simulink library "tenneco_lib"  (R2016b)
settings: Solver=ode45  StartTime=0.0  StopTime=10.0  RelTol=1e-3
undefined symbols (not defined in the file): Com_cntAMBInitTO_c, Com_cntAMBStopTO_c, Com_cntEC1InitTO_c, Com_cntEC1StopTO_c, Com_swAMBRx_c, Com_swEC1Rx_c, Com_swUseSPN108_c, Com_swUseSPN543_c, const, Env_pAmbPDflt_c, Env_pAmbPKOff_c, Env_pAmbPOvrd_c, Env_swAmbPOvrd_c, MSG_INIT_TIMEOUT, MSG_NOT_RECEIVED, MSG_RECEIVED_NOW, MSG_STOP_TIMEOUT
libraries: simulink x19, tenneco_lib x2
(part 5 of 5)

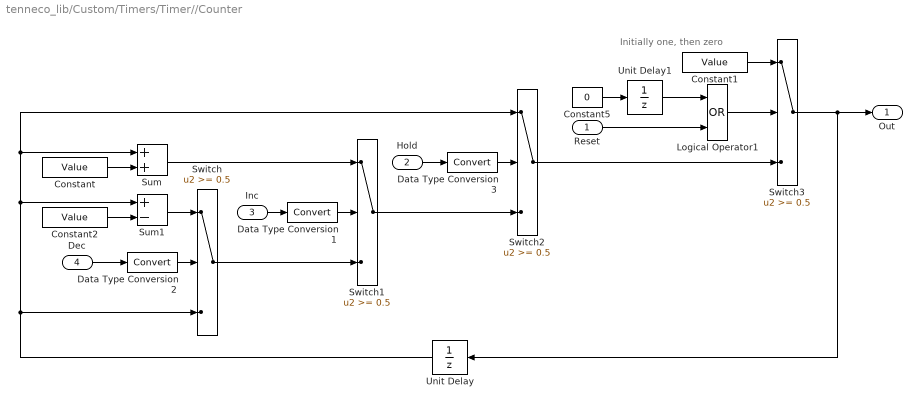
== system tenneco_lib/Custom/Timers/Timer//Counter ==
  note: Initially one,
      | then zero
  Reset : Inport  mask(Standard Inport){Port=1}
      mask prompts: Port "Simulink:blkprm_prompts:InOutportPortNum"
      mask help: Provide an input port for subsystems.
      mask TypeOptions Port: Port
  Hold : Inport  Port=2  mask(Standard Inport){Port=2}
      mask prompts: Port "Simulink:blkprm_prompts:InOutportPortNum"
      mask help: Provide an input port for subsystems.
      mask TypeOptions Port: Port
  Inc : Inport  Port=3  mask(Standard Inport){Port=3}
      mask prompts: Port "Simulink:blkprm_prompts:InOutportPortNum"
      mask help: Provide an input port for subsystems.
      mask TypeOptions Port: Port
  Dec : Inport  Port=4  mask(Standard Inport){Port=4}
      mask prompts: Port "Simulink:blkprm_prompts:InOutportPortNum"
      mask help: Provide an input port for subsystems.
      mask TypeOptions Port: Port
  Constant : Constant  Value=Value  mask(Constant){Value=INC_STEP}
      mask prompts: Value "Simulink:blkprm_prompts:ConstConstValue"
      mask help: Output the constant specified by the 'Constant value' parameter. If 'Constant value' is a vector, treat the constant value as a 1-D array.
      mask init: same as tenneco_lib/Custom/Logical/Latch/Constant
      mask TypeOptions Value: Value
      mask Display: disp(str)
  Constant1 : Constant  Value=Value  mask(Constant){Value=INIT}
      mask prompts: Value "Simulink:blkprm_prompts:ConstConstValue"
      mask help: Output the constant specified by the 'Constant value' parameter. If 'Constant value' is a vector, treat the constant value as a 1-D array.
      mask init: same as tenneco_lib/Custom/Logical/Latch/Constant
      mask TypeOptions Value: Value
      mask Display: disp(str)
  Constant2 : Constant  Value=Value  mask(Constant){Value=DEC_STEP}
      mask prompts: Value "Simulink:blkprm_prompts:ConstConstValue"
      mask help: Output the constant specified by the 'Constant value' parameter. If 'Constant value' is a vector, treat the constant value as a 1-D array.
      mask init: same as tenneco_lib/Custom/Logical/Latch/Constant
      mask TypeOptions Value: Value
      mask Display: disp(str)
  Constant5 : Constant  Value=0  OutDataTypeStr=Inherit: Inherit via back propagation
  Data Type Conversion1 : DataTypeConversion  mask(Data Type Conversion){OutDataTypeStr=Inherit: Inherit via back propagation}
      mask prompts: OutDataTypeStr "Simulink:blkprm_prompts:OUTPUT_UNIFIEDDATATYPE"
      mask help: Convert the input to the data type and scaling of the output.
      mask TypeOptions OutDataTypeStr: OutDataTypeStr
  Data Type Conversion2 : DataTypeConversion  mask(Data Type Conversion){OutDataTypeStr=Inherit: Inherit via back propagation}
      mask prompts: OutDataTypeStr "Simulink:blkprm_prompts:OUTPUT_UNIFIEDDATATYPE"
      mask help: Convert the input to the data type and scaling of the output.
      mask TypeOptions OutDataTypeStr: OutDataTypeStr
  Data Type Conversion3 : DataTypeConversion  mask(Data Type Conversion){OutDataTypeStr=Inherit: Inherit via back propagation}
      mask prompts: OutDataTypeStr "Simulink:blkprm_prompts:OUTPUT_UNIFIEDDATATYPE"
      mask help: Convert the input to the data type and scaling of the output.
      mask TypeOptions OutDataTypeStr: OutDataTypeStr
  Logical Operator1 : Logic  Operator=OR  Inputs=Inputs  AllPortsSameDT=off  OutDataTypeStr=boolean  mask(Logical Operator){Operator=OR, Inputs=2}
      mask prompts: Operator "Simulink:blkprm_prompts:LogicOperator"; Inputs "Simulink:blkprm_prompts:LogicNumInputPorts"
      mask help: Logical operators. For a single input, operators are applied across the input vector. For multiple inputs, operators are applied across the inputs.
      mask TypeOptions Operator: Operator
      mask TypeOptions Inputs: Inputs
  Sum : Sum  InputSameDT=on  mask(Sum){Inputs=++}
      mask prompts: Inputs "Simulink:blkprm_prompts:SumListofSigns"
      mask help:
      | Add or subtract inputs.  Specify one of the following:
      | a) character vector containing + or - for each input port, | for spacer between ports (e.g. ++|-|++)
      | b) scalar, >= 1, specifies the number of input ports to be summed.
      | When there is only one input port, add or subtract elements over all dimensions or one specified dimension
      mask TypeOptions Inputs: Inputs
  Sum1 : Sum  Inputs=+-  InputSameDT=on  mask(Sum){Inputs=+-}
      mask prompts: Inputs "Simulink:blkprm_prompts:SumListofSigns"
      mask help:
      | Add or subtract inputs.  Specify one of the following:
      | a) character vector containing + or - for each input port, | for spacer between ports (e.g. ++|-|++)
      | b) scalar, >= 1, specifies the number of input ports to be summed.
      | When there is only one input port, add or subtract elements over all dimensions or one specified dimension
      mask TypeOptions Inputs: Inputs
  Switch : Switch  Threshold=0.5  mask(Switch){}
      mask help: Pass through input 1 when input 2 satisfies the selected criterion; otherwise, pass through input 3. The inputs are numbered top to bottom (or left to right). The first and third input ports are data ports, and the second input port is the control port. The criteria for control port 2 are u2 >= Threshold (0.5).
  Switch1 : Switch  Threshold=0.5  mask(Switch){}
      mask help: Pass through input 1 when input 2 satisfies the selected criterion; otherwise, pass through input 3. The inputs are numbered top to bottom (or left to right). The first and third input ports are data ports, and the second input port is the control port. The criteria for control port 2 are u2 >= Threshold (0.5).
  Switch2 : Switch  Threshold=0.5  mask(Switch){}
      mask help: Pass through input 1 when input 2 satisfies the selected criterion; otherwise, pass through input 3. The inputs are numbered top to bottom (or left to right). The first and third input ports are data ports, and the second input port is the control port. The criteria for control port 2 are u2 >= Threshold (0.5).
  Switch3 : Switch  Threshold=0.5  mask(Switch){}
      mask help: Pass through input 1 when input 2 satisfies the selected criterion; otherwise, pass through input 3. The inputs are numbered top to bottom (or left to right). The first and third input ports are data ports, and the second input port is the control port. The criteria for control port 2 are u2 >= Threshold (0.5).
  Unit Delay : UnitDelay  InitialCondition=InitialCondition  SampleTime=-1  mask(Unit Delay){InitialCondition=0}
      mask prompts: InitialCondition "Simulink:blkprm_prompts:DelayBlkInitCond"
      mask help: Sample and hold with one sample period delay.
      mask TypeOptions InitialCondition: InitialCondition
  Unit Delay1 : UnitDelay  InitialCondition=InitialCondition  SampleTime=-1  mask(Unit Delay){InitialCondition=0}
      mask prompts: InitialCondition "Simulink:blkprm_prompts:DelayBlkInitCond"
      mask help: Sample and hold with one sample period delay.
      mask TypeOptions InitialCondition: InitialCondition
  Out : Outport  mask(Standard Outport){Port=1}
      mask prompts: Port "Simulink:blkprm_prompts:InOutportPortNum"
      mask help: Provide an output port for subsystems.
      mask TypeOptions Port: Port
  wires:
  Data Type Conversion3/1 -> Switch2/2
  Data Type Conversion2/1 -> Switch/2
  Data Type Conversion1/1 -> Switch1/2
  Reset/1 -> Logical Operator1/2
  Unit Delay1/1 -> Logical Operator1/1
  Logical Operator1/1 -> Switch3/2
  Hold/1 -> Data Type Conversion3/1
  Switch2/1 -> Switch3/3
  Switch1/1 -> Switch2/3
  Constant2/1 -> Sum1/2
  Constant/1 -> Sum/2
  Switch3/1 -> Out/1, Unit Delay/1
  Sum1/1 -> Switch/1
  Sum/1 -> Switch1/1
  Switch/1 -> Switch1/3
  Unit Delay/1 -> Switch/3, Sum/1, Switch2/1, Sum1/1
  Dec/1 -> Data Type Conversion2/1
  Inc/1 -> Data Type Conversion1/1
  Constant5/1 -> Unit Delay1/1
  Constant1/1 -> Switch3/1

== system tenneco_lib/Model Documentation/Appendix Title/Description1 ==
  DocBlock : simulink/Model-Wide Utilities/DocBlock  DocumentType=RTF

== system tenneco_lib/ButterWorth Filters/Generic Low-Pass Filter/Stabilize Counter/Increment Counter ==
  note: Note : Simulink constant block used because Tenneco constant block is not generic and datatype friendly
  x : Inport  mask(Standard Inport){Port=1}
      mask prompts: Port "Simulink:blkprm_prompts:InOutportPortNum"
      mask help: Provide an input port for subsystems.
      mask TypeOptions Port: Port
  Enable : EnablePort  StatesWhenEnabling=reset  mask(Enable Port){StatesWhenEnabling=reset, ShowOutputPort=off}
      mask prompts: StatesWhenEnabling "Simulink:blkprm_prompts:EnabPortStates"; ShowOutputPort "Simulink:blkprm_prompts:TrigEnabShowOutPort"
      mask help: Place this block in a subsystem or at the root level of a model to create an enabled system.
      mask TypeOptions StatesWhenEnabling: StatesWhenEnabling
      mask TypeOptions ShowOutputPort: ShowOutputPort
  Constant9 : Constant  OutDataTypeStr=Inherit: Inherit via back propagation
  Sum : Sum  InputSameDT=on  mask(Sum){Inputs=++}
      mask prompts: Inputs "Simulink:blkprm_prompts:SumListofSigns"
      mask help:
      | Add or subtract inputs.  Specify one of the following:
      | a) character vector containing + or - for each input port, | for spacer between ports (e.g. ++|-|++)
      | b) scalar, >= 1, specifies the number of input ports to be summed.
      | When there is only one input port, add or subtract elements over all dimensions or one specified dimension
      mask TypeOptions Inputs: Inputs
  x+1 : Outport  mask(Standard Outport){Port=1}
      mask prompts: Port "Simulink:blkprm_prompts:InOutportPortNum"
      mask help: Provide an output port for subsystems.
      mask TypeOptions Port: Port
  wires:
  Sum/1 -> x+1/1
  x/1 -> Sum/2
  Constant9/1 -> Sum/1

== system tenneco_lib/ButterWorth Filters/Resettable Variable Low-Pass Filter/Stabilize Counter/Increment Counter ==
  x : Inport  mask(Standard Inport){Port=1}
      mask prompts: Port "Simulink:blkprm_prompts:InOutportPortNum"
      mask help: Provide an input port for subsystems.
      mask TypeOptions Port: Port
  Enable : EnablePort  mask(Enable Port){StatesWhenEnabling=held, ShowOutputPort=off}
      mask prompts: StatesWhenEnabling "Simulink:blkprm_prompts:EnabPortStates"; ShowOutputPort "Simulink:blkprm_prompts:TrigEnabShowOutPort"
      mask help: Place this block in a subsystem or at the root level of a model to create an enabled system.
      mask TypeOptions StatesWhenEnabling: StatesWhenEnabling
      mask TypeOptions ShowOutputPort: ShowOutputPort
  Constant9 : Constant  OutDataTypeStr=Inherit: Inherit via back propagation
  Sum : Sum  InputSameDT=on  mask(Sum){Inputs=++}
      mask prompts: Inputs "Simulink:blkprm_prompts:SumListofSigns"
      mask help:
      | Add or subtract inputs.  Specify one of the following:
      | a) character vector containing + or - for each input port, | for spacer between ports (e.g. ++|-|++)
      | b) scalar, >= 1, specifies the number of input ports to be summed.
      | When there is only one input port, add or subtract elements over all dimensions or one specified dimension
      mask TypeOptions Inputs: Inputs
  x+1 : Outport  mask(Standard Outport){Port=1}
      mask prompts: Port "Simulink:blkprm_prompts:InOutportPortNum"
      mask help: Provide an output port for subsystems.
      mask TypeOptions Port: Port
  wires:
  Sum/1 -> x+1/1
  x/1 -> Sum/2
  Constant9/1 -> Sum/1

== system tenneco_lib/ButterWorth Filters/Variable Low-Pass Filter/Stabilize Counter/Increment Counter ==
  x : Inport  mask(Standard Inport){Port=1}
      mask prompts: Port "Simulink:blkprm_prompts:InOutportPortNum"
      mask help: Provide an input port for subsystems.
      mask TypeOptions Port: Port
  Enable : EnablePort  mask(Enable Port){StatesWhenEnabling=held, ShowOutputPort=off}
      mask prompts: StatesWhenEnabling "Simulink:blkprm_prompts:EnabPortStates"; ShowOutputPort "Simulink:blkprm_prompts:TrigEnabShowOutPort"
      mask help: Place this block in a subsystem or at the root level of a model to create an enabled system.
      mask TypeOptions StatesWhenEnabling: StatesWhenEnabling
      mask TypeOptions ShowOutputPort: ShowOutputPort
  Constant9 : Constant  OutDataTypeStr=Inherit: Inherit via back propagation
  Sum : Sum  InputSameDT=on  mask(Sum){Inputs=++}
      mask prompts: Inputs "Simulink:blkprm_prompts:SumListofSigns"
      mask help:
      | Add or subtract inputs.  Specify one of the following:
      | a) character vector containing + or - for each input port, | for spacer between ports (e.g. ++|-|++)
      | b) scalar, >= 1, specifies the number of input ports to be summed.
      | When there is only one input port, add or subtract elements over all dimensions or one specified dimension
      mask TypeOptions Inputs: Inputs
  x+1 : Outport  mask(Standard Outport){Port=1}
      mask prompts: Port "Simulink:blkprm_prompts:InOutportPortNum"
      mask help: Provide an output port for subsystems.
      mask TypeOptions Port: Port
  wires:
  Sum/1 -> x+1/1
  x/1 -> Sum/2
  Constant9/1 -> Sum/1

== system tenneco_lib/Custom/CAN/Generic CAN Input/Timeout Check ==
  CAN_RX : Inport  mask(Standard Inport){Port=1}
      mask prompts: Port "Simulink:blkprm_prompts:InOutportPortNum"
      mask help: Provide an input port for subsystems.
      mask TypeOptions Port: Port
  Eng_stIgn : Inport  Port=2  mask(Standard Inport){Port=2}
      mask prompts: Port "Simulink:blkprm_prompts:InOutportPortNum"
      mask help: Provide an input port for subsystems.
      mask TypeOptions Port: Port
  Constant : Constant  Value=Value  mask(Constant){Value=CAN_CNT_INIT}
      mask prompts: Value "Simulink:blkprm_prompts:ConstConstValue"
      mask help: Output the constant specified by the 'Constant value' parameter. If 'Constant value' is a vector, treat the constant value as a 1-D array.
      mask init: same as tenneco_lib/Sources/Constant
      mask TypeOptions Value: Value
      mask Display: disp(str)
  Constant1 : Constant  Value=Value  mask(Constant){Value=CAN_CNT_STOP}
      mask prompts: Value "Simulink:blkprm_prompts:ConstConstValue"
      mask help: Output the constant specified by the 'Constant value' parameter. If 'Constant value' is a vector, treat the constant value as a 1-D array.
      mask init: same as tenneco_lib/Sources/Constant
      mask TypeOptions Value: Value
      mask Display: disp(str)
  Timeout Check : tenneco_lib/Custom/CAN/Timeout Check
  CAN_TO : Outport  mask(Standard Outport){Port=1}
      mask prompts: Port "Simulink:blkprm_prompts:InOutportPortNum"
      mask help: Provide an output port for subsystems.
      mask TypeOptions Port: Port
  wires:
  CAN_RX/1 -> Timeout Check/1
  Constant1/1 -> Timeout Check/4
  Constant/1 -> Timeout Check/3
  Eng_stIgn/1 -> Timeout Check/2
  Timeout Check/1 -> CAN_TO/1

== system tenneco_lib/Custom/CAN/Generic Valueless CAN Input/Timeout Check ==
  CAN_RX : Inport  mask(Standard Inport){Port=1}
      mask prompts: Port "Simulink:blkprm_prompts:InOutportPortNum"
      mask help: Provide an input port for subsystems.
      mask TypeOptions Port: Port
  Eng_stIgn : Inport  Port=2  mask(Standard Inport){Port=2}
      mask prompts: Port "Simulink:blkprm_prompts:InOutportPortNum"
      mask help: Provide an input port for subsystems.
      mask TypeOptions Port: Port
  Constant2 : Constant  Value=Value  mask(Constant){Value=CAN_CNT_INIT}
      mask prompts: Value "Simulink:blkprm_prompts:ConstConstValue"
      mask help: Output the constant specified by the 'Constant value' parameter. If 'Constant value' is a vector, treat the constant value as a 1-D array.
      mask init: same as tenneco_lib/Sources/Constant
      mask TypeOptions Value: Value
      mask Display: disp(str)
  Constant3 : Constant  Value=Value  mask(Constant){Value=CAN_CNT_STOP}
      mask prompts: Value "Simulink:blkprm_prompts:ConstConstValue"
      mask help: Output the constant specified by the 'Constant value' parameter. If 'Constant value' is a vector, treat the constant value as a 1-D array.
      mask init: same as tenneco_lib/Sources/Constant
      mask TypeOptions Value: Value
      mask Display: disp(str)
  Timeout Check : tenneco_lib/Custom/CAN/Timeout Check
  CAN_TO : Outport  mask(Standard Outport){Port=1}
      mask prompts: Port "Simulink:blkprm_prompts:InOutportPortNum"
      mask help: Provide an output port for subsystems.
      mask TypeOptions Port: Port
  wires:
  Eng_stIgn/1 -> Timeout Check/2
  CAN_RX/1 -> Timeout Check/1
  Constant2/1 -> Timeout Check/3
  Constant3/1 -> Timeout Check/4
  Timeout Check/1 -> CAN_TO/1

== system tenneco_lib/Custom/CAN/Timeout Check/Timeout Check ==
  note: Should not reach this state
  note: Message timeout
      | without receive
  note: Message not yet
      | received once, but
      | not yet timed out
  Input Signal : Inport  mask(Standard Inport){Port=1}
      mask prompts: Port "Simulink:blkprm_prompts:InOutportPortNum"
      mask help: Provide an input port for subsystems.
      mask TypeOptions Port: Port
  Init Timeout Limit : Inport  Port=2  mask(Standard Inport){Port=2}
      mask prompts: Port "Simulink:blkprm_prompts:InOutportPortNum"
      mask help: Provide an input port for subsystems.
      mask TypeOptions Port: Port
  Stop Timeout Limit : Inport  Port=3  mask(Standard Inport){Port=3}
      mask prompts: Port "Simulink:blkprm_prompts:InOutportPortNum"
      mask help: Provide an input port for subsystems.
      mask TypeOptions Port: Port
  Enable : EnablePort  StatesWhenEnabling=reset  mask(Enable Port){StatesWhenEnabling=reset, ShowOutputPort=off}
      mask prompts: StatesWhenEnabling "Simulink:blkprm_prompts:EnabPortStates"; ShowOutputPort "Simulink:blkprm_prompts:TrigEnabShowOutPort"
      mask help: Place this block in a subsystem or at the root level of a model to create an enabled system.
      mask TypeOptions StatesWhenEnabling: StatesWhenEnabling
      mask TypeOptions ShowOutputPort: ShowOutputPort
  Constant : Constant  Value=Value  mask(Constant){Value=MSG_NOT_RECEIVED}
      mask prompts: Value "Simulink:blkprm_prompts:ConstConstValue"
      mask help: Output the constant specified by the 'Constant value' parameter. If 'Constant value' is a vector, treat the constant value as a 1-D array.
      mask init: same as tenneco_lib/Sources/Constant
      mask TypeOptions Value: Value
      mask Display: disp(str)
  Constant1 : Constant  Value=Value  mask(Constant){Value=MSG_NOT_RECEIVED}
      mask prompts: Value "Simulink:blkprm_prompts:ConstConstValue"
      mask help: Output the constant specified by the 'Constant value' parameter. If 'Constant value' is a vector, treat the constant value as a 1-D array.
      mask init: same as tenneco_lib/Sources/Constant
      mask TypeOptions Value: Value
      mask Display: disp(str)
  Constant2 : Constant  Value=Value  mask(Constant){Value=MSG_INIT_TIMEOUT}
      mask prompts: Value "Simulink:blkprm_prompts:ConstConstValue"
      mask help: Output the constant specified by the 'Constant value' parameter. If 'Constant value' is a vector, treat the constant value as a 1-D array.
      mask init: same as tenneco_lib/Sources/Constant
      mask TypeOptions Value: Value
      mask Display: disp(str)
  Initial Timeout Check : Subsystem
  Logical Operator : Logic  Operator=OR  Inputs=Inputs  AllPortsSameDT=off  OutDataTypeStr=boolean  mask(Logical Operator){Operator=OR, Inputs=2}
      mask prompts: Operator "Simulink:blkprm_prompts:LogicOperator"; Inputs "Simulink:blkprm_prompts:LogicNumInputPorts"
      mask help: Logical operators. For a single input, operators are applied across the input vector. For multiple inputs, operators are applied across the inputs.
      mask TypeOptions Operator: Operator
      mask TypeOptions Inputs: Inputs
  Missing Count : Subsystem
  Stop Timeout Check : Subsystem
  Switch : Switch  Threshold=0.5  mask(Switch){}
      mask help: Pass through input 1 when input 2 satisfies the selected criterion; otherwise, pass through input 3. The inputs are numbered top to bottom (or left to right). The first and third input ports are data ports, and the second input port is the control port. The criteria for control port 2 are u2 >= Threshold (0.5).
  Switch1 : Switch  Threshold=0.5  mask(Switch){}
      mask help: Pass through input 1 when input 2 satisfies the selected criterion; otherwise, pass through input 3. The inputs are numbered top to bottom (or left to right). The first and third input ports are data ports, and the second input port is the control port. The criteria for control port 2 are u2 >= Threshold (0.5).
  Switch2 : Switch  Threshold=0.5  mask(Switch){}
      mask help: Pass through input 1 when input 2 satisfies the selected criterion; otherwise, pass through input 3. The inputs are numbered top to bottom (or left to right). The first and third input ports are data ports, and the second input port is the control port. The criteria for control port 2 are u2 >= Threshold (0.5).
  Unit Delay1 : UnitDelay  InitialCondition=InitialCondition  SampleTime=-1  mask(Unit Delay){InitialCondition=0}
      mask prompts: InitialCondition "Simulink:blkprm_prompts:DelayBlkInitCond"
      mask help: Sample and hold with one sample period delay.
      mask TypeOptions InitialCondition: InitialCondition
  Timeout Code : Outport  mask(Standard Outport){Port=1}
      mask prompts: Port "Simulink:blkprm_prompts:InOutportPortNum"
      mask help: Provide an output port for subsystems.
      mask TypeOptions Port: Port
  wires:
  Switch1/1 -> Switch2/1
  Initial Timeout Check/1(Init Timeout) -> Switch1/2, Switch/2
  Constant2/1 -> Switch/1
  Switch/1 -> Switch2/3
  Missing Count/1(Missing Count) -> Stop Timeout Check/1(Missing Count), Initial Timeout Check/1(Missing Count)
  Constant/1 -> Switch/3
  Input Signal/1 -> Logical Operator/1, Initial Timeout Check/2(Input Signal), Missing Count/1(Input Signal)
  Switch2/1 -> Timeout Code/1
  Unit Delay1/1 -> Logical Operator/2
  Logical Operator/1 -> Switch2/2, Unit Delay1/1
  Init Timeout Limit/1 -> Initial Timeout Check/3(Init Timeout Limit)
  Stop Timeout Limit/1 -> Stop Timeout Check/2(StopTimeout Limit)
  Constant1/1 -> Switch1/1
  [stop_timeout] -> Switch1/3
  Stop Timeout Check/1(Stop Timeout) -> [stop_timeout]

== system tenneco_lib/Custom/Math/Divide by zero protection/If Action Subsystem1 ==
  In1 : Inport  mask(Standard Inport){Port=1}
      mask prompts: Port "Simulink:blkprm_prompts:InOutportPortNum"
      mask help: Provide an input port for subsystems.
      mask TypeOptions Port: Port
  In2 : Inport  Port=2  mask(Standard Inport){Port=2}
      mask prompts: Port "Simulink:blkprm_prompts:InOutportPortNum"
      mask help: Provide an input port for subsystems.
      mask TypeOptions Port: Port
  Action Port : ActionPort
  Product : Product  Inputs=*/  InputSameDT=on  mask(Product){Inputs=*/}
      mask prompts: Inputs "List of signs:"
      mask help:
      | Multiply or divide inputs.  Specify one of the following:
      |  a) * or / for each input port. For example, **/* performs the operation 'u1*u2/u3*u4'.
      |  b) scalar specifies the number of input ports to be multiplied.
      mask TypeOptions Inputs: Inputs
  Out1 : Outport  mask(Standard Outport){Port=1}
      mask prompts: Port "Simulink:blkprm_prompts:InOutportPortNum"
      mask help: Provide an output port for subsystems.
      mask TypeOptions Port: Port
  wires:
  Product/1 -> Out1/1
  In1/1 -> Product/1
  In2/1 -> Product/2

== system tenneco_lib/Custom/Math/Divide by zero protection/If Action Subsystem2 ==
  Action Port : ActionPort
  Constant : Constant  Value=Value  mask(Constant){Value=default}
      mask prompts: Value "Simulink:blkprm_prompts:ConstConstValue"
      mask help: Output the constant specified by the 'Constant value' parameter. If 'Constant value' is a vector, treat the constant value as a 1-D array.
      mask init: same as tenneco_lib/Custom/Logical/Latch/Constant
      mask TypeOptions Value: Value
      mask Display: disp(str)
  Out1 : Outport  mask(Standard Outport){Port=1}
      mask prompts: Port "Simulink:blkprm_prompts:InOutportPortNum"
      mask help: Provide an output port for subsystems.
      mask TypeOptions Port: Port
  wires:
  Constant/1 -> Out1/1

== system tenneco_lib/Custom/Math/Time_Based_Rate_Limiter/First_Order_System ==
  Input : Inport  mask(Standard Inport){Port=1}
      mask prompts: Port "Simulink:blkprm_prompts:InOutportPortNum"
      mask help: Provide an input port for subsystems.
      mask TypeOptions Port: Port
  Tau : Inport  Port=2  mask(Standard Inport){Port=2}
      mask prompts: Port "Simulink:blkprm_prompts:InOutportPortNum"
      mask help: Provide an input port for subsystems.
      mask TypeOptions Port: Port
  Constant1 : Constant  OutDataTypeStr=Inherit: Inherit via back propagation
  Constant3 : Constant  OutDataTypeStr=Inherit: Inherit via back propagation
  Constant4 : Constant  Value=2*Fs  OutDataTypeStr=Inherit: Inherit via back propagation
  Product1 : Product  Inputs=*/  InputSameDT=on  mask(Product){Inputs=*/}
      mask prompts: Inputs "List of signs:"
      mask help:
      | Multiply or divide inputs.  Specify one of the following:
      |  a) * or / for each input port. For example, **/* performs the operation 'u1*u2/u3*u4'.
      |  b) scalar specifies the number of input ports to be multiplied.
      mask TypeOptions Inputs: Inputs
  Product2 : Product  Inputs=**  InputSameDT=on  mask(Product){Inputs=**}
      mask prompts: Inputs "List of signs:"
      mask help:
      | Multiply or divide inputs.  Specify one of the following:
      |  a) * or / for each input port. For example, **/* performs the operation 'u1*u2/u3*u4'.
      |  b) scalar specifies the number of input ports to be multiplied.
      mask TypeOptions Inputs: Inputs
  Product3 : Product  Inputs=**  InputSameDT=on  mask(Product){Inputs=**}
      mask prompts: Inputs "List of signs:"
      mask help:
      | Multiply or divide inputs.  Specify one of the following:
      |  a) * or / for each input port. For example, **/* performs the operation 'u1*u2/u3*u4'.
      |  b) scalar specifies the number of input ports to be multiplied.
      mask TypeOptions Inputs: Inputs
  Sum : Sum  Inputs=+-  InputSameDT=on  mask(Sum){Inputs=+-}
      mask prompts: Inputs "Simulink:blkprm_prompts:SumListofSigns"
      mask help:
      | Add or subtract inputs.  Specify one of the following:
      | a) character vector containing + or - for each input port, | for spacer between ports (e.g. ++|-|++)
      | b) scalar, >= 1, specifies the number of input ports to be summed.
      | When there is only one input port, add or subtract elements over all dimensions or one specified dimension
      mask TypeOptions Inputs: Inputs
  Sum1 : Sum  InputSameDT=on  mask(Sum){Inputs=++}
      mask prompts: Inputs "Simulink:blkprm_prompts:SumListofSigns"
      mask help:
      | Add or subtract inputs.  Specify one of the following:
      | a) character vector containing + or - for each input port, | for spacer between ports (e.g. ++|-|++)
      | b) scalar, >= 1, specifies the number of input ports to be summed.
      | When there is only one input port, add or subtract elements over all dimensions or one specified dimension
      mask TypeOptions Inputs: Inputs
  Sum2 : Sum  Inputs=-+  InputSameDT=on  mask(Sum){Inputs=-+}
      mask prompts: Inputs "Simulink:blkprm_prompts:SumListofSigns"
      mask help:
      | Add or subtract inputs.  Specify one of the following:
      | a) character vector containing + or - for each input port, | for spacer between ports (e.g. ++|-|++)
      | b) scalar, >= 1, specifies the number of input ports to be summed.
      | When there is only one input port, add or subtract elements over all dimensions or one specified dimension
      mask TypeOptions Inputs: Inputs
  Sum3 : Sum  InputSameDT=on  mask(Sum){Inputs=++}
      mask prompts: Inputs "Simulink:blkprm_prompts:SumListofSigns"
      mask help:
      | Add or subtract inputs.  Specify one of the following:
      | a) character vector containing + or - for each input port, | for spacer between ports (e.g. ++|-|++)
      | b) scalar, >= 1, specifies the number of input ports to be summed.
      | When there is only one input port, add or subtract elements over all dimensions or one specified dimension
      mask TypeOptions Inputs: Inputs
  Unit Delay : UnitDelay  InitialCondition=InitialCondition  SampleTime=-1  mask(Unit Delay){InitialCondition=0}
      mask prompts: InitialCondition "Simulink:blkprm_prompts:DelayBlkInitCond"
      mask help: Sample and hold with one sample period delay.
      mask TypeOptions InitialCondition: InitialCondition
  Unit Delay1 : UnitDelay  InitialCondition=InitialCondition  SampleTime=-1  mask(Unit Delay){InitialCondition=0}
      mask prompts: InitialCondition "Simulink:blkprm_prompts:DelayBlkInitCond"
      mask help: Sample and hold with one sample period delay.
      mask TypeOptions InitialCondition: InitialCondition
  Output : Outport  mask(Standard Outport){Port=1}
      mask prompts: Port "Simulink:blkprm_prompts:InOutportPortNum"
      mask help: Provide an output port for subsystems.
      mask TypeOptions Port: Port
  wires:
  Constant3/1 -> Sum1/2
  Constant1/1 -> Sum2/1
  [Inp] -> Sum3/2
  Product1/1 -> Product2/2
  Sum1/1 -> Product1/2
  Sum2/1 -> Product1/1
  Product3/1 -> Sum2/2, Sum1/1
  Constant4/1 -> Product3/2
  Tau/1 -> Product3/1
  Sum3/1 -> Output/1, Unit Delay1/1
  Product2/1 -> Sum3/1
  Sum/1 -> Product2/1
  Unit Delay1/1 -> Sum/1
  Unit Delay/1 -> Sum/2, [Inp]
  Input/1 -> Unit Delay/1

== system tenneco_lib/Custom/CAN/Timeout Check/Timeout Check/Initial Timeout Check ==
  Missing Count : Inport  mask(Standard Inport){Port=1}
      mask prompts: Port "Simulink:blkprm_prompts:InOutportPortNum"
      mask help: Provide an input port for subsystems.
      mask TypeOptions Port: Port
  Input Signal : Inport  Port=2  mask(Standard Inport){Port=2}
      mask prompts: Port "Simulink:blkprm_prompts:InOutportPortNum"
      mask help: Provide an input port for subsystems.
      mask TypeOptions Port: Port
  Init Timeout Limit : Inport  Port=3  mask(Standard Inport){Port=3}
      mask prompts: Port "Simulink:blkprm_prompts:InOutportPortNum"
      mask help: Provide an input port for subsystems.
      mask TypeOptions Port: Port
  Logical Operator1 : Logic  Operator=OR  Inputs=Inputs  AllPortsSameDT=off  OutDataTypeStr=boolean  mask(Logical Operator){Operator=OR, Inputs=2}
      mask prompts: Operator "Simulink:blkprm_prompts:LogicOperator"; Inputs "Simulink:blkprm_prompts:LogicNumInputPorts"
      mask help: Logical operators. For a single input, operators are applied across the input vector. For multiple inputs, operators are applied across the inputs.
      mask TypeOptions Operator: Operator
      mask TypeOptions Inputs: Inputs
  Logical Operator3 : Logic  Inputs=Inputs  AllPortsSameDT=off  OutDataTypeStr=boolean  mask(Logical Operator){Operator=AND, Inputs=2}
      mask prompts: Operator "Simulink:blkprm_prompts:LogicOperator"; Inputs "Simulink:blkprm_prompts:LogicNumInputPorts"
      mask help: Logical operators. For a single input, operators are applied across the input vector. For multiple inputs, operators are applied across the inputs.
      mask TypeOptions Operator: Operator
      mask TypeOptions Inputs: Inputs
  Logical Operator4 : Logic  Operator=NOT  Inputs=Inputs  AllPortsSameDT=off  OutDataTypeStr=boolean  mask(Logical Operator){Operator=NOT, Inputs=2}
      mask prompts: Operator "Simulink:blkprm_prompts:LogicOperator"; Inputs "Simulink:blkprm_prompts:LogicNumInputPorts"
      mask help: Logical operators. For a single input, operators are applied across the input vector. For multiple inputs, operators are applied across the inputs.
      mask TypeOptions Operator: Operator
      mask TypeOptions Inputs: Inputs
  Relational Operator : RelationalOperator  Operator=>  OutDataTypeStr=boolean  RndMeth=Nearest  mask(Relational Operator){Operator=>}
      mask prompts: Operator "Simulink:blkprm_prompts:RelopOperator"
      mask help: Applies the selected relational operator to the inputs and outputs the result. The top (or left) input corresponds to the first operand.
      mask TypeOptions Operator: Operator
  Unit Delay2 : UnitDelay  InitialCondition=InitialCondition  SampleTime=-1  mask(Unit Delay){InitialCondition=0}
      mask prompts: InitialCondition "Simulink:blkprm_prompts:DelayBlkInitCond"
      mask help: Sample and hold with one sample period delay.
      mask TypeOptions InitialCondition: InitialCondition
  Init Timeout : Outport  mask(Standard Outport){Port=1}
      mask prompts: Port "Simulink:blkprm_prompts:InOutportPortNum"
      mask help: Provide an output port for subsystems.
      mask TypeOptions Port: Port
  wires:
  Missing Count/1 -> Relational Operator/1
  Relational Operator/1 -> Logical Operator3/1
  Unit Delay2/1 -> Logical Operator1/2
  Logical Operator1/1 -> Unit Delay2/1, Logical Operator4/1
  Logical Operator3/1 -> Init Timeout/1
  Init Timeout Limit/1 -> Relational Operator/2
  Logical Operator4/1 -> Logical Operator3/2
  Input Signal/1 -> Logical Operator1/1

== system tenneco_lib/Custom/CAN/Timeout Check/Timeout Check/Missing Count ==
  note: Note : Simulink constant block used because Tenneco constant block is not generic and datatype friendly
  Input Signal : Inport  mask(Standard Inport){Port=1}
      mask prompts: Port "Simulink:blkprm_prompts:InOutportPortNum"
      mask help: Provide an input port for subsystems.
      mask TypeOptions Port: Port
  Constant1 : Constant  OutDataTypeStr=Inherit: Inherit via back propagation
  Constant5 : Constant  Value=0  OutDataTypeStr=Inherit: Inherit via back propagation
  Logical Operator1 : Logic  Operator=NOT  Inputs=Inputs  AllPortsSameDT=off  OutDataTypeStr=boolean  mask(Logical Operator){Operator=NOT, Inputs=2}
      mask prompts: Operator "Simulink:blkprm_prompts:LogicOperator"; Inputs "Simulink:blkprm_prompts:LogicNumInputPorts"
      mask help: Logical operators. For a single input, operators are applied across the input vector. For multiple inputs, operators are applied across the inputs.
      mask TypeOptions Operator: Operator
      mask TypeOptions Inputs: Inputs
  Sum1 : Sum  InputSameDT=on  mask(Sum){Inputs=++}
      mask prompts: Inputs "Simulink:blkprm_prompts:SumListofSigns"
      mask help:
      | Add or subtract inputs.  Specify one of the following:
      | a) character vector containing + or - for each input port, | for spacer between ports (e.g. ++|-|++)
      | b) scalar, >= 1, specifies the number of input ports to be summed.
      | When there is only one input port, add or subtract elements over all dimensions or one specified dimension
      mask TypeOptions Inputs: Inputs
  Switch1 : Switch  Threshold=0.5  mask(Switch){}
      mask help: Pass through input 1 when input 2 satisfies the selected criterion; otherwise, pass through input 3. The inputs are numbered top to bottom (or left to right). The first and third input ports are data ports, and the second input port is the control port. The criteria for control port 2 are u2 >= Threshold (0.5).
  Unit Delay1 : UnitDelay  InitialCondition=InitialCondition  SampleTime=-1  mask(Unit Delay){InitialCondition=0}
      mask prompts: InitialCondition "Simulink:blkprm_prompts:DelayBlkInitCond"
      mask help: Sample and hold with one sample period delay.
      mask TypeOptions InitialCondition: InitialCondition
  Missing Count : Outport  mask(Standard Outport){Port=1}
      mask prompts: Port "Simulink:blkprm_prompts:InOutportPortNum"
      mask help: Provide an output port for subsystems.
      mask TypeOptions Port: Port
  wires:
  Constant5/1 -> Switch1/3
  Logical Operator1/1 -> Switch1/2
  Input Signal/1 -> Logical Operator1/1
  Constant1/1 -> Sum1/2
  Unit Delay1/1 -> Sum1/1
  Sum1/1 -> Switch1/1
  Switch1/1 -> Missing Count/1, Unit Delay1/1

== system tenneco_lib/Custom/CAN/Timeout Check/Timeout Check/Stop Timeout Check ==
  note: Message timeout
      | after initially received
  note: Message ok
  Missing Count : Inport  mask(Standard Inport){Port=1}
      mask prompts: Port "Simulink:blkprm_prompts:InOutportPortNum"
      mask help: Provide an input port for subsystems.
      mask TypeOptions Port: Port
  StopTimeout Limit : Inport  Port=2  mask(Standard Inport){Port=2}
      mask prompts: Port "Simulink:blkprm_prompts:InOutportPortNum"
      mask help: Provide an input port for subsystems.
      mask TypeOptions Port: Port
  Constant3 : Constant  Value=Value  mask(Constant){Value=MSG_STOP_TIMEOUT}
      mask prompts: Value "Simulink:blkprm_prompts:ConstConstValue"
      mask help: Output the constant specified by the 'Constant value' parameter. If 'Constant value' is a vector, treat the constant value as a 1-D array.
      mask init: same as tenneco_lib/Sources/Constant
      mask TypeOptions Value: Value
      mask Display: disp(str)
  Constant4 : Constant  Value=Value  mask(Constant){Value=MSG_RECEIVED_NOW}
      mask prompts: Value "Simulink:blkprm_prompts:ConstConstValue"
      mask help: Output the constant specified by the 'Constant value' parameter. If 'Constant value' is a vector, treat the constant value as a 1-D array.
      mask init: same as tenneco_lib/Sources/Constant
      mask TypeOptions Value: Value
      mask Display: disp(str)
  Relational Operator : RelationalOperator  Operator=>  OutDataTypeStr=boolean  RndMeth=Nearest  mask(Relational Operator){Operator=>}
      mask prompts: Operator "Simulink:blkprm_prompts:RelopOperator"
      mask help: Applies the selected relational operator to the inputs and outputs the result. The top (or left) input corresponds to the first operand.
      mask TypeOptions Operator: Operator
  Switch1 : Switch  Threshold=0.5  mask(Switch){}
      mask help: Pass through input 1 when input 2 satisfies the selected criterion; otherwise, pass through input 3. The inputs are numbered top to bottom (or left to right). The first and third input ports are data ports, and the second input port is the control port. The criteria for control port 2 are u2 >= Threshold (0.5).
  Stop Timeout : Outport  mask(Standard Outport){Port=1}
      mask prompts: Port "Simulink:blkprm_prompts:InOutportPortNum"
      mask help: Provide an output port for subsystems.
      mask TypeOptions Port: Port
  wires:
  Switch1/1 -> Stop Timeout/1
  Constant4/1 -> Switch1/3
  Constant3/1 -> Switch1/1
  StopTimeout Limit/1 -> Relational Operator/2
  Missing Count/1 -> Relational Operator/1
  Relational Operator/1 -> Switch1/2
